simulink model "CoffeeReactor_ex2_linear_discrete"  (R2023b)
settings: Solver=ode4  StartTime=0.0  StopTime=simulationParameters.Tsim  FixedStep=simulationParameters.Tint  RelTol=1e-3
undefined symbols (not defined in the file): simulationParameters, sys_d
settings Model: Creator=simone  LastModifiedBy=fabiomosele
settings SolverCC: AlgebraicLoopSolver=TrustRegion
settings DataIOCC: SaveOutput=off  SignalLogging=off  DSMLogging=off  SaveTime=off  ReturnWorkspaceOutputs=off
settings DebuggingCC: UnconnectedInputMsg=warning  UnconnectedOutputMsg=warning  UnconnectedLineMsg=warning
settings ModelReferenceCC: EnableRefExpFcnMdlSchedulingChecks=on
settings RTWCC: DLArmComputeVersion=19.05

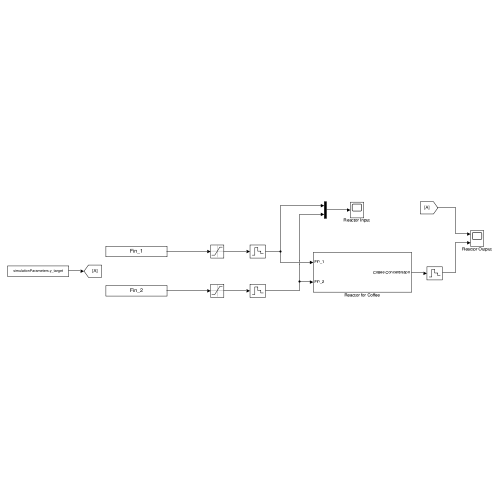
[thumbnail: Simulink's stored preview of the top-level diagram]
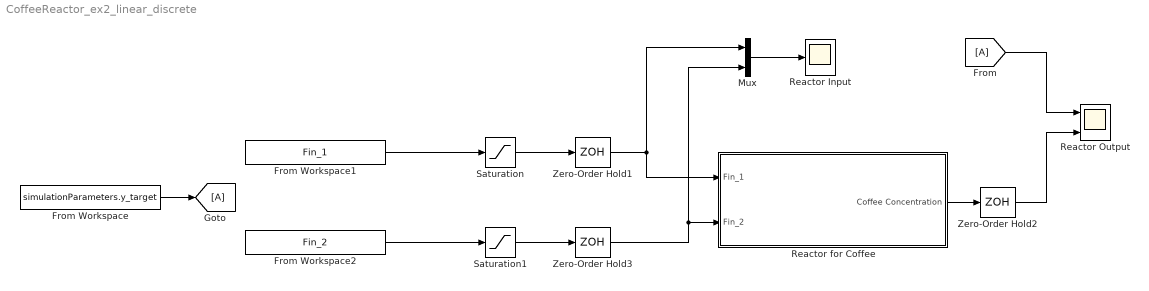
== system CoffeeReactor_ex2_linear_discrete ==
  From : From
  From Workspace : FromWorkspace  VariableName=simulationParameters.y_target  OutputAfterFinalValue=Holding final value
  From Workspace1 : FromWorkspace  VariableName=Fin_1  OutputAfterFinalValue=Holding final value
  From Workspace2 : FromWorkspace  VariableName=Fin_2  OutputAfterFinalValue=Holding final value
  Goto : Goto
  Mux : Mux  Inputs=2
  Reactor Input : Scope
  Reactor Output : Scope  NumInputPorts=2
  Reactor for Coffee : Subsystem
  Saturation : Saturate  UpperLimit=simulationParameters.Fin1_max  LowerLimit=simulationParameters.Fin1_min
  Saturation1 : Saturate  UpperLimit=simulationParameters.Fin2_max  LowerLimit=simulationParameters.Fin2_min
  Zero-Order Hold1 : ZeroOrderHold  SampleTime=simulationParameters.Ts
  Zero-Order Hold2 : ZeroOrderHold  SampleTime=simulationParameters.Ts
  Zero-Order Hold3 : ZeroOrderHold  SampleTime=simulationParameters.Ts
  wires:
  Reactor for Coffee/1(Coffee Concentration) -> Zero-Order Hold2/1
  Zero-Order Hold2/1 -> Reactor Output/2
  From/1 -> Reactor Output/1
  Mux/1 -> Reactor Input/1
  From Workspace2/1 -> Saturation1/1
  From Workspace1/1 -> Saturation/1
  Zero-Order Hold1/1 -> Reactor for Coffee/1(Fin_1), Mux/1
  Zero-Order Hold3/1 -> Reactor for Coffee/2(Fin_2), Mux/2
  Saturation/1 -> Zero-Order Hold1/1
  Saturation1/1 -> Zero-Order Hold3/1
  From Workspace/1 -> Goto/1

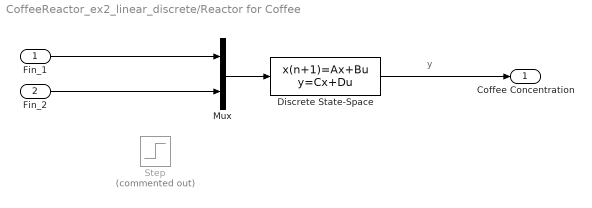
== system CoffeeReactor_ex2_linear_discrete/Reactor for Coffee ==
  note: y
  Fin_1 : Inport
  Fin_2 : Inport  Port=2
  Discrete State-Space : DiscreteStateSpace  A=sys_d.A  B=sys_d.B  C=sys_d.C  D=sys_d.D  InitialCondition=simulationParameters.Reactor_parameters.x_0  SampleTime=-1
  Mux : Mux  Inputs=2
  Step : Step  Commented=on  Time=simulationParameters.Reactor_parameters.Tdist  After=simulationParameters.Reactor_parameters.Adist  SampleTime=0
  Coffee Concentration : Outport
  wires:
  Fin_2/1 -> Mux/2
  Fin_1/1 -> Mux/1
  Mux/1 -> Discrete State-Space/1
  Discrete State-Space/1 -> Coffee Concentration/1
